simulink model "simpletest1"  (R2024a)
settings: Solver=VariableStepAuto  StartTime=0.0  StopTime=10.0  RelTol=1e-3
undefined symbols (not defined in the file): pino, prova1
libraries: hdlBasic x4, vmcUtilities x1
settings Model: Creator=valbas  LastModifiedBy=valbas

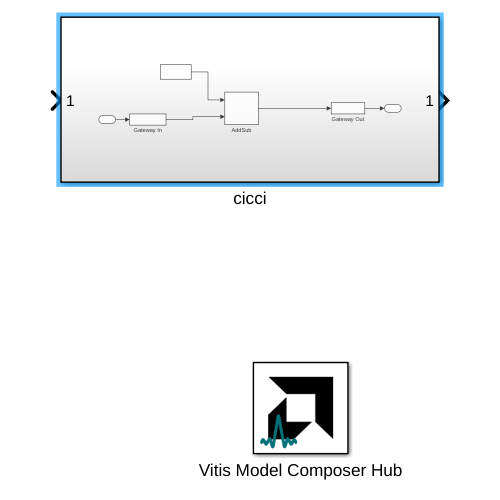
[thumbnail: Simulink's stored preview of the top-level diagram]
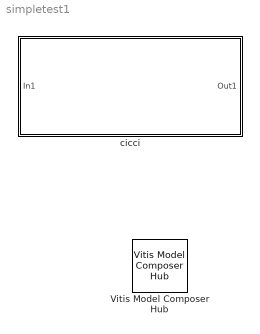
== system simpletest1 ==
  Vitis Model Composer Hub : vmcUtilities/Vitis Model Composer Hub  Tag=genX  CodeGeneration=off  SubsystemName=pino  BlockHierPath=prova1/pino  CompilationType=HDLCompilation  SubsystemType=HDLNode  ExportTypeV2=IP Catalog  StartColumn=1  NumberOfColumns=1  TargetDirectory=./netlist/ip/pino/src  exportDesign=on  analyzeDesign=off  validateDesignOnHw=off  ExportType=AI Engines  IpVendor=xilinx.com  IpLibrary=hls  IpVersion=1.0  IpHWLanguage=Verilog  AieCompilerOptions={}  AieSimulatorOptions={}  CreateTestbench=off  TestbenchStackSize=10  RunRtlSim=off  RunCSim=off  RunAieSim=off  AieSimTimeout=50000  RunAieSimProfiling=off  LaunchVitisAnalyzer=off  PlotOutput=off  RunX86Sim=off  X86SimTimeout=10  GenHwImage=off  GenLibadfXo=on  GenHwValidationCode=off  PlatformType=Not Specified  HwSystemType=Baremetal  HwValidationTarget=hw  ProjDevice=Zynq UltraScale+ ZCU106 Evaluation Platform (xczu7ev-ffvc1156-2-e)  ProjDevicePart=xczu7ev-ffvc1156-2-e  AIEType=None  SamplePeriod=-1  ClockFrequency=200  DataPathParallelism=1  directory=./netlist/ip/pino/src  testbench=off  incr_netlist=off  synthesis_tool=Vivado  clock_wrapper=Clock Enables  dbl_ovrd=According to Block Masks  dcm_input_clock_period=10  sysclk_period=8  simulink_period=8.e-9  eval_field=0  IPInfoJsonString="{\"DUTSubsystemName\":\"pino\",\"HDLSubsystem\":{\"SubsystemName\":\"pino\",\"IPName\":\"Subsystem\",\"IPLibrary\":\"VMC\",\"IPVendor\":\"User Company\",\"IPVersion\":\"1.0\",\"TargetDirectory\":\"./netlist\",\"SubsystemDir\":\"./netlist/ip/pino\",\"FreqHz\":\"125000000\"},\"SubsystemTag\":\"HDLNode\"}"  LogFileName=/xilinxworks/ZCU106/v2025.2/chopsync/gitcode/modelcomp/netlist/model_composer.log  NThreads=4  IPConfigFile=/tmp/vmctmp-5005312303136637390/prova1_ipconfig.json
  cicci : Subsystem

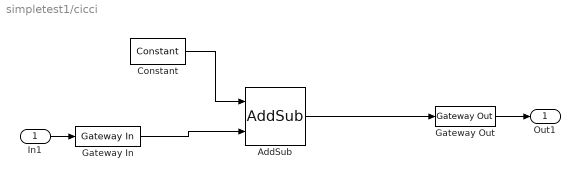
== system simpletest1/cicci ==
  In1 : Inport
  AddSub : hdlBasic/AddSub  mode=Addition  use_carryin=off  use_carryout=off  en=off  latency=1  precision=Full  arith_type=Unsigned  n_bits=16  bin_pt=14  quantization=Truncate  overflow=Wrap  use_behavioral_HDL=off  hw_selection=Fabric  pipelined=off  XmcBlockStatus=1  maskContainerNames=tabcontainer1  block_type=addsub  block_config=sysgen:Addsub_config
  Constant : hdlBasic/Constant  const=1.0  gui_display_data_type=Fixed-point  arith_type=Signed (2's comp)  n_bits=16  bin_pt=14  preci_type=Single  exp_width=8  frac_width=24  explicit_period=off  period=1  XmcBlockStatus=1  maskContainerNames=tabcontainer1  block_type=constant  block_config=sysgen:Constant_config
  Gateway In : hdlBasic/Gateway In  gui_display_data_type=Fixed-point  arith_type=Signed (2's comp)  n_bits=16  bin_pt=14  preci_type=Single  exp_width=8  frac_width=24  rows=1  columns=1  quantization="Round  (unbiased: +/- Inf)"  overflow=Saturate  period=1  UseAsADC=off  ADCChannel='1'  interface=None  automatic_assignment=on  address_offset=hex2dec('00')  intf_name=''  intf_description=''  default_value=0  timing_constraint=None  locs_specified=off  LOCs={}  io_standard={}  inherit_from_input=off  hdl_port=on  XmcBlockStatus=1  maskContainerNames=group4  block_type=gatewayin  block_config=sysgen:gateway_in_config  block_width_w=590  block_height_w=620  block_width=640  block_height=850
  Gateway Out : hdlBasic/Gateway Out  inherit_from_input=off  bool_to_boolean=off  hdl_port=on  rows=1  columns=1  UseAsDAC=off  DACChannel='1'  interface=None  automatic_assignment=on  address_offset=hex2dec('00')  intf_name=''  intf_description=''  timing_constraint=None  locs_specified=off  LOCs={}  io_standard={}  XmcBlockStatus=1  maskContainerNames=group4  block_type=gatewayout  block_config=sysgen:gateway_out_config  block_width_w=590  block_height_w=620  block_width=620  block_height=750
  Out1 : Outport
  wires:
  Constant/1 -> AddSub/1
  Gateway In/1 -> AddSub/2
  AddSub/1 -> Gateway Out/1
  Gateway Out/1 -> Out1/1
  In1/1 -> Gateway In/1
